simulink model "fwr1_org"  (Simulink 10.0)
settings: Solver=ode45  StartTime=0.0  StopTime=2  RelTol=1e-3  EnableMultiTasking=on
settings Model: Creator=omar  LastModifiedBy=annonymous
settings DataIOCC: LimitDataPoints=on
settings DebuggingCC: UnderspecifiedInitializationDetection=Simplified  MergeDetectMultiDrivingBlocksExec=error
settings GRTTargetCC: GeneratePreprocessorConditionals=Disable all  CombineOutputUpdateFcns=on  GRTInterface=off
settings ConfigComp: CovExternalEMLEnable=off

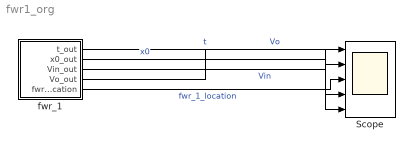
== system fwr1_org ==
  Scope : Scope  NumInputPorts=5
  fwr_1 : Stateflow chart  TreatAsAtomicUnit=on
  wires:
  fwr_1/4(Vo_out) -> Scope/1  "Vo"
  fwr_1/1(t_out) -> Scope/2  "t"
  fwr_1/5(fwr_1_location) -> Scope/3  "fwr_1_location"
  fwr_1/3(Vin_out) -> Scope/4  "Vin"
  fwr_1/2(x0_out) -> Scope/5  "x0"

== stateflow chart fwr_1 ==
  settings: updateMethod=CONTINUOUS
  state D1_on
    du:
    t_dot = 1;
    x0_dot = Vin;
    Vin_dot = -x0 * (2 * pi * f) ^ 2;
    Vo_dot = Vin / Rd * C - Vo * (1 / Rd * C + 1 / R * C);
    t_out=t;
    x0_out=x0;
    Vin_out=Vin;
    Vo_out=Vo;
    fwr_1_location =1;
  state D2_on
    du:
    t_dot = 1;
    x0_dot = Vin;
    Vin_dot = -x0 * (2 * pi * f) ^ 2;
    Vo_dot = -Vin / Rd * C - Vo * (1 / Rd * C + 1 / R * C);
    t_out=t;
    x0_out=x0;
    Vin_out=Vin;
    Vo_out=Vo;
    fwr_1_location =2;
  state both_off
    du:
    t_dot = 1;
    x0_dot = Vin;
    Vin_dot = -x0 * (2 * pi * f) ^ 2;
    Vo_dot = -Vo / R * C;
    t_out=t;
    x0_out=x0;
    Vin_out=Vin;
    Vo_out=Vo;
    fwr_1_location =3;
  both_off -> D1_on [order 1] : [Vin >= Vo && -Vin <= Vo]
      | {t = t;}
  D1_on -> D2_on [order 1] : [Vin <= Vo]
      | {t = t;}
  D2_on -> D1_on [order 1] : [Vin >= Vo]
      | {t = t;}
  (default) -> D1_on : {t = 0;
      | x0 = -0.012738853503184714;
      | Vin = 4;
      | Vo = 4;}
  D1_on -> both_off [order 2] : [Vin <= Vo && -Vin <= Vo]
      | {t = t;}
  both_off -> D2_on [order 2] : [Vin <= Vo && -Vin >= Vo]
      | {t = t;}
  D2_on -> both_off [order 2] : [Vin <= Vo && -Vin <= Vo]
      | {t = t;}
  data: t_out output double; t local double; x0_out output double; x0 local double; Vin_out output double; Vin local double; Vo_out output double; Vo local double; fwr_1_location output double; f constant double =50; tmax constant double =2; Rd constant double =0.1; Vmax constant double =4; R constant double =1000; C constant double =0.0001; pi constant double =3.14
  data t settings: updateMethod=SF_CONTINUOUS_TIME_DATA
  data x0 settings: updateMethod=SF_CONTINUOUS_TIME_DATA
  data Vin settings: updateMethod=SF_CONTINUOUS_TIME_DATA
  data Vo settings: updateMethod=SF_CONTINUOUS_TIME_DATA
